simulink model "PassiveHydPTO_Version_3"  (R2014a)
settings: Solver=ode23tb  StartTime=0.0  StopTime=param.stop  FixedStep=0.01  MaxStep=0.05  RelTol=1e-6
values from neighbouring files (symbols this model uses):
  alpha = 1    [Main.m]
  Amax = 0.001    [Main.m]
  Amin = 1e-8    (= 1e-08)    [Main.m]
  Ap = 2.35e-2    (= 0.0235)    [Main.m]
  Beta_e = 1.86e9    (= 1860000000)    [Main.m]
  bf = 0.05*bg    (= 0.118735)    [Main.m]
  bg = 2.3747    [Main.m]
  Cd = 0.61    [Main.m]
  D = 3.9789e-5    (= 3.9789e-05)    [Main.m]
  f = 1/period    (= 0.1)    [Main.m]
  J = 3.961    [Main.m]
  k1 = 200    [Main.m]
  k2 = atanh((Amin-(Amax-Amin)/2)*      2/(Amax - Amin))*1/(pMin-(pMax + pMin)/2)    [Main.m]
  omega_i = 0    [Main.m]
  pAeq = pCeq    (= 21333333.3333)    [Main.m]
  pAi = pAeq    (= 21333333.3333)    [Main.m]
  pAupper_limit = 32e6    (= 32000000)    [Main.m]
  pBeq = pCeq    (= 21333333.3333)    [Main.m]
  pBi = pBeq    (= 21333333.3333)    [Main.m]
  pBupper_limit = 32e6    (= 32000000)    [Main.m]
  pCprecharge = 0.9*pClower_limit    (= 19200000)    [Main.m]
  pDprecharge = 0.9*pDlower_limit    (= 9600000)    [Main.m]
  pMax = 1e6    (= 1000000)    [Main.m]
  pMin = 0.75e6    (= 750000)    [Main.m]
  rho = 850    [Main.m]
  VC0 = 7.5    [Main.m]
  VCeq = VC0*(1-(pCprecharge/pCeq)^(1/1.4))    (= 0.543715404282)    [Main.m]
  VD0 = 3    [Main.m]
  VDeq = VDmax    (= 1.30403881906)    [Main.m]
  Vo = Ap*5    (= 0.1175)    [Main.m]
settings Model: Creator=sor  LastModifiedBy=sor

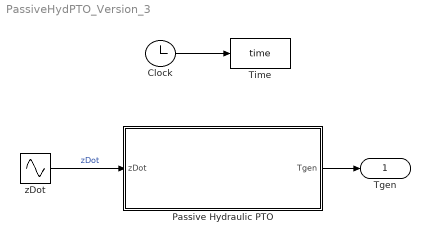
== system PassiveHydPTO_Version_3 ==
  Clock : Clock
  "Passive Hydraulic PTO " : Subsystem
  Time : ToWorkspace  VariableName=time  SampleTime=-1
  zDot : Sin  Amplitude=0.8  Frequency=2*pi*f  SampleTime=0
  Tgen : Outport
  wires:
  Clock/1 -> Time/1
  zDot/1 -> "Passive Hydraulic PTO "/1(zDot)  "zDot"
  "Passive Hydraulic PTO "/1(Tgen) -> Tgen/1

== system PassiveHydPTO_Version_3/Passive Hydraulic PTO  ==
  zDot : Inport
  High Pressure Accumulator : Subsystem
  Low Pressure Accumulator : Subsystem
  Motor Generator : Subsystem
  "Piston Pump " : Subsystem
  Rectified Valve : Subsystem
  Tgen : Outport
  wires:
  "Piston Pump "/1(pA) -> Rectified Valve/1(pA)
  Motor Generator/1(Tgen) -> Tgen/1
  High Pressure Accumulator/1(pC) -> Motor Generator/1(pC), Rectified Valve/3(pC)  "pC"
  Low Pressure Accumulator/1(pD) -> Rectified Valve/4(pD), Motor Generator/2(pD)  "pD"
  "Piston Pump "/2(pB) -> Rectified Valve/2(pB)
  zDot/1 -> "Piston Pump "/1(zDot)
  Rectified Valve/1(Vdot) -> Low Pressure Accumulator/1(Vdot), High Pressure Accumulator/1(Vdot), "Piston Pump "/2(Vdot)
  Motor Generator/2(omega) -> Low Pressure Accumulator/2(omega), High Pressure Accumulator/2(omega)

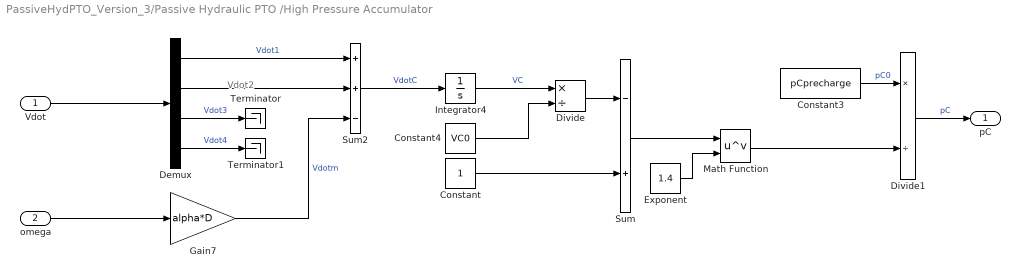
== system PassiveHydPTO_Version_3/Passive Hydraulic PTO /High Pressure Accumulator ==
  note: Vdot2
  Vdot : Inport
  omega : Inport  Port=2
  Constant : Constant
  Constant3 : Constant  Value=pCprecharge
  Constant4 : Constant  Value=VC0
  Demux : Demux
  Divide : Product  Inputs=*/
  Divide1 : Product  Inputs=*/
  Exponent : Constant  Value=1.4
  Gain7 : Gain  Gain=alpha*D
  Integrator4 : Integrator  InitialCondition=VCeq
  Math Function : Math  Operator=pow  SaturateOnIntegerOverflow=on
  Sum : Sum  Inputs=-+
  Sum2 : Sum  Inputs=++-
  Terminator : Terminator
  Terminator1 : Terminator
  pC : Outport
  wires:
  Sum2/1 -> Integrator4/1  "VdotC"
  Integrator4/1 -> Divide/1  "VC"
  Constant4/1 -> Divide/2
  Constant/1 -> Sum/2
  Divide/1 -> Sum/1
  Exponent/1 -> Math Function/2
  Sum/1 -> Math Function/1
  Math Function/1 -> Divide1/2
  Constant3/1 -> Divide1/1  "pC0"
  Divide1/1 -> pC/1  "pC"
  Vdot/1 -> Demux/1
  Demux/3 -> Terminator/1  "Vdot3"
  Demux/4 -> Terminator1/1  "Vdot4"
  omega/1 -> Gain7/1
  Demux/1 -> Sum2/1  "Vdot1"
  Demux/2 -> Sum2/2
  Gain7/1 -> Sum2/3  "Vdotm"

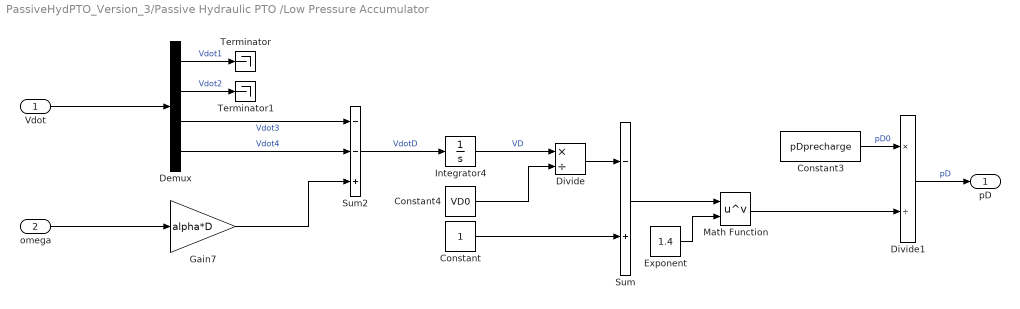
== system PassiveHydPTO_Version_3/Passive Hydraulic PTO /Low Pressure Accumulator ==
  Vdot : Inport
  omega : Inport  Port=2
  Constant : Constant
  Constant3 : Constant  Value=pDprecharge
  Constant4 : Constant  Value=VD0
  Demux : Demux
  Divide : Product  Inputs=*/
  Divide1 : Product  Inputs=*/
  Exponent : Constant  Value=1.4
  Gain7 : Gain  Gain=alpha*D
  Integrator4 : Integrator  InitialCondition=VDeq
  Math Function : Math  Operator=pow  SaturateOnIntegerOverflow=on
  Sum : Sum  Inputs=-+
  Sum2 : Sum  Inputs=--+
  Terminator : Terminator
  Terminator1 : Terminator
  pD : Outport
  wires:
  Sum2/1 -> Integrator4/1  "VdotD"
  Integrator4/1 -> Divide/1  "VD"
  Constant4/1 -> Divide/2
  Constant/1 -> Sum/2
  Divide/1 -> Sum/1
  Exponent/1 -> Math Function/2
  Sum/1 -> Math Function/1
  Math Function/1 -> Divide1/2
  Constant3/1 -> Divide1/1  "pD0"
  Divide1/1 -> pD/1  "pD"
  Vdot/1 -> Demux/1
  Demux/3 -> Sum2/1  "Vdot3"
  Demux/4 -> Sum2/2  "Vdot4"
  omega/1 -> Gain7/1
  Gain7/1 -> Sum2/3
  Demux/1 -> Terminator/1  "Vdot1"
  Demux/2 -> Terminator1/1  "Vdot2"

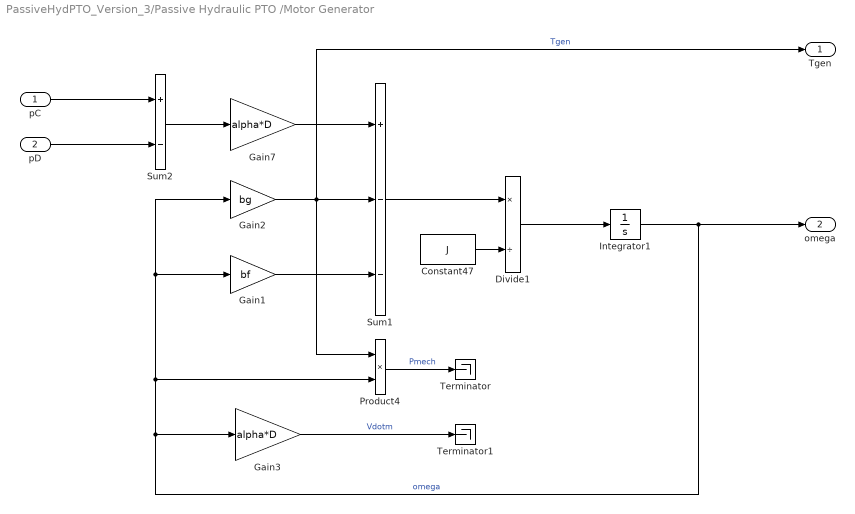
== system PassiveHydPTO_Version_3/Passive Hydraulic PTO /Motor Generator ==
  pC : Inport
  pD : Inport  Port=2
  Constant47 : Constant  Value=J
  Divide1 : Product  Inputs=*/
  Gain1 : Gain  Gain=bf
  Gain2 : Gain  Gain=bg
  Gain3 : Gain  Gain=alpha*D
  Gain7 : Gain  Gain=alpha*D
  Integrator1 : Integrator  InitialCondition=omega_i
  Product4 : Product
  Sum1 : Sum  Inputs=+--
  Sum2 : Sum  Inputs=+-
  Terminator : Terminator
  Terminator1 : Terminator
  Tgen : Outport
  omega : Outport  Port=2
  wires:
  pC/1 -> Sum2/1
  pD/1 -> Sum2/2
  Sum2/1 -> Gain7/1
  Gain7/1 -> Sum1/1
  Gain2/1 -> Product4/1, Tgen/1, Sum1/2  "Tgen"
  Gain1/1 -> Sum1/3
  Sum1/1 -> Divide1/1
  Constant47/1 -> Divide1/2
  Product4/1 -> Terminator/1  "Pmech"
  Divide1/1 -> Integrator1/1
  Integrator1/1 -> Gain3/1, Gain1/1, Gain2/1, Product4/2, omega/1  "omega"
  Gain3/1 -> Terminator1/1  "Vdotm"

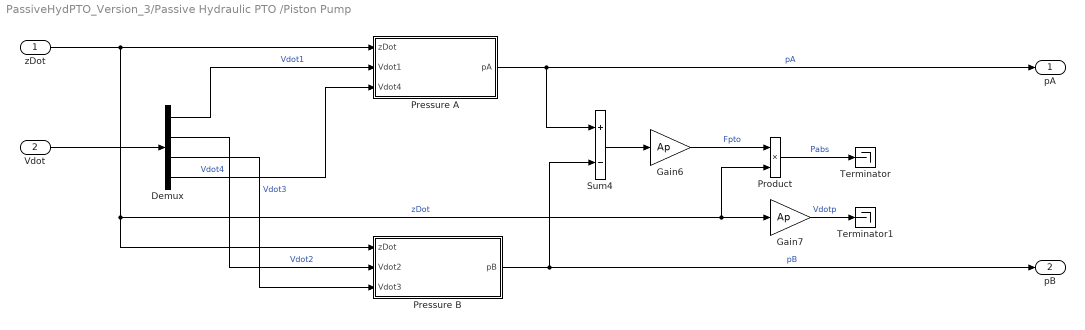
== system PassiveHydPTO_Version_3/Passive Hydraulic PTO /Piston Pump  ==
  zDot : Inport
  Vdot : Inport  Port=2
  Demux : Demux
  Gain6 : Gain  Gain=Ap
  Gain7 : Gain  Gain=Ap
  Pressure A : Subsystem
  Pressure B : Subsystem
  Product : Product
  Sum4 : Sum  Inputs=+-
  Terminator : Terminator
  Terminator1 : Terminator
  pA : Outport
  pB : Outport  Port=2
  wires:
  Pressure A/1(pA) -> pA/1, Sum4/1  "pA"
  Pressure B/1(pB) -> Sum4/2, pB/1  "pB"
  Gain7/1 -> Terminator1/1  "Vdotp"
  Gain6/1 -> Product/1  "Fpto"
  Product/1 -> Terminator/1  "Pabs"
  Vdot/1 -> Demux/1
  zDot/1 -> Gain7/1, Product/2, Pressure B/1(zDot), Pressure A/1(zDot)  "zDot"
  Demux/1 -> Pressure A/2(Vdot1)  "Vdot1"
  Demux/2 -> Pressure B/2(Vdot2)  "Vdot2"
  Demux/3 -> Pressure B/3(Vdot3)  "Vdot3"
  Demux/4 -> Pressure A/3(Vdot4)  "Vdot4"
  Sum4/1 -> Gain6/1

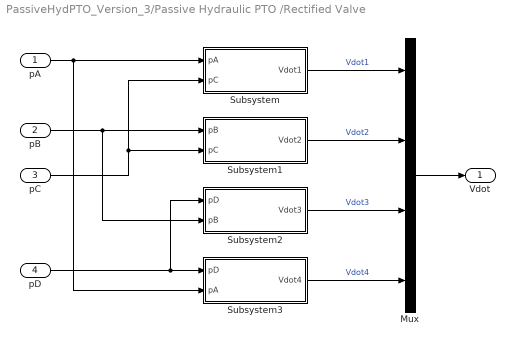
== system PassiveHydPTO_Version_3/Passive Hydraulic PTO /Rectified Valve ==
  pA : Inport
  pB : Inport  Port=2
  pC : Inport  Port=3
  pD : Inport  Port=4
  Mux : Mux
  Subsystem : Subsystem
  Subsystem1 : Subsystem
  Subsystem2 : Subsystem
  Subsystem3 : Subsystem
  Vdot : Outport
  wires:
  pA/1 -> Subsystem3/2(pA), Subsystem/1(pA)
  pB/1 -> Subsystem2/2(pB), Subsystem1/1(pB)
  pC/1 -> Subsystem1/2(pC), Subsystem/2(pC)
  pD/1 -> Subsystem3/1(pD), Subsystem2/1(pD)
  Subsystem3/1(Vdot4) -> Mux/4  "Vdot4"
  Subsystem2/1(Vdot3) -> Mux/3  "Vdot3"
  Subsystem1/1(Vdot2) -> Mux/2  "Vdot2"
  Subsystem/1(Vdot1) -> Mux/1  "Vdot1"
  Mux/1 -> Vdot/1

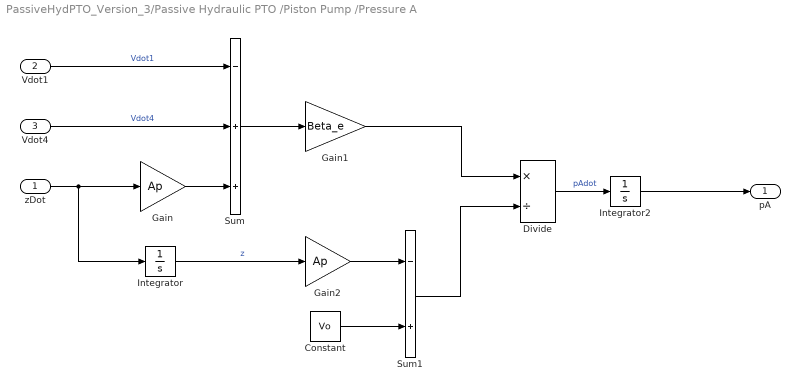
== system PassiveHydPTO_Version_3/Passive Hydraulic PTO /Piston Pump /Pressure A ==
  zDot : Inport
  Vdot1 : Inport  Port=2
  Vdot4 : Inport  Port=3
  Constant : Constant  Value=Vo
  Divide : Product  Inputs=*/
  Gain : Gain  Gain=Ap
  Gain1 : Gain  Gain=Beta_e
  Gain2 : Gain  Gain=Ap
  Integrator : Integrator
  Integrator2 : Integrator  InitialCondition=pAi  UpperSaturationLimit=pAupper_limit  LowerSaturationLimit=pAeq
  Sum : Sum  Inputs=-++
  Sum1 : Sum  Inputs=-+
  pA : Outport
  wires:
  Gain/1 -> Sum/3
  Sum/1 -> Gain1/1
  zDot/1 -> Integrator/1, Gain/1
  Integrator/1 -> Gain2/1  "z"
  Gain2/1 -> Sum1/1
  Constant/1 -> Sum1/2
  Gain1/1 -> Divide/1
  Sum1/1 -> Divide/2
  Vdot1/1 -> Sum/1  "Vdot1"
  Divide/1 -> Integrator2/1  "pAdot"
  Vdot4/1 -> Sum/2  "Vdot4"
  Integrator2/1 -> pA/1

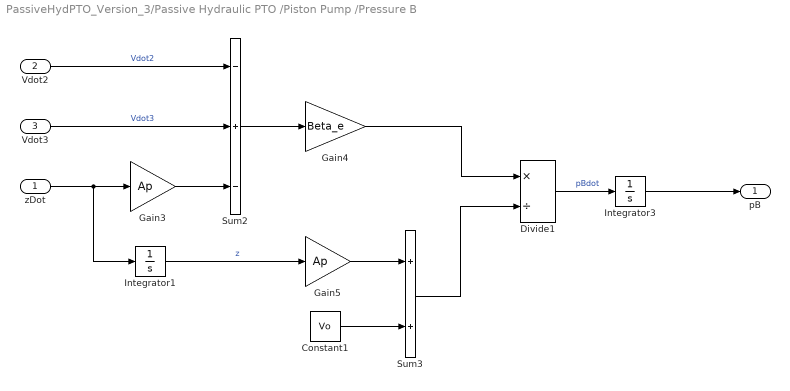
== system PassiveHydPTO_Version_3/Passive Hydraulic PTO /Piston Pump /Pressure B ==
  zDot : Inport
  Vdot2 : Inport  Port=2
  Vdot3 : Inport  Port=3
  Constant1 : Constant  Value=Vo
  Divide1 : Product  Inputs=*/
  Gain3 : Gain  Gain=Ap
  Gain4 : Gain  Gain=Beta_e
  Gain5 : Gain  Gain=Ap
  Integrator1 : Integrator
  Integrator3 : Integrator  InitialCondition=pBi  UpperSaturationLimit=pBupper_limit  LowerSaturationLimit=pBeq
  Sum2 : Sum  Inputs=-+-
  Sum3 : Sum
  pB : Outport
  wires:
  Gain3/1 -> Sum2/3
  Sum2/1 -> Gain4/1
  zDot/1 -> Integrator1/1, Gain3/1
  Integrator1/1 -> Gain5/1  "z"
  Gain5/1 -> Sum3/1
  Constant1/1 -> Sum3/2
  Gain4/1 -> Divide1/1
  Sum3/1 -> Divide1/2
  Divide1/1 -> Integrator3/1  "pBdot"
  Vdot2/1 -> Sum2/1  "Vdot2"
  Vdot3/1 -> Sum2/2  "Vdot3"
  Integrator3/1 -> pB/1

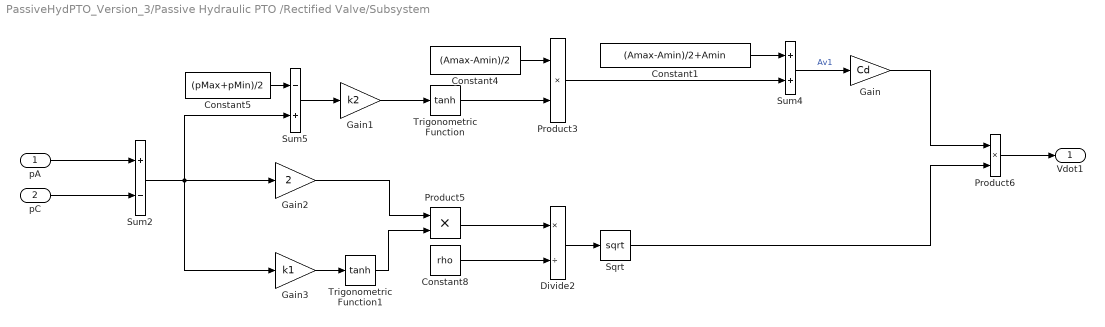
== system PassiveHydPTO_Version_3/Passive Hydraulic PTO /Rectified Valve/Subsystem ==
  pA : Inport
  pC : Inport  Port=2
  Constant1 : Constant  Value=(Amax-Amin)/2+Amin
  Constant4 : Constant  Value=(Amax-Amin)/2
  Constant5 : Constant  Value=(pMax+pMin)/2
  Constant8 : Constant  Value=rho
  Divide2 : Product  Inputs=*/
  Gain : Gain  Gain=Cd
  Gain1 : Gain  Gain=k2
  Gain2 : Gain  Gain=2
  Gain3 : Gain  Gain=k1
  Product3 : Product
  Product5 : Product
  Product6 : Product
  Sqrt : Sqrt  SaturateOnIntegerOverflow=on
  Sum2 : Sum  Inputs=+-
  Sum4 : Sum
  Sum5 : Sum  Inputs=-+
  Trigonometric Function : Trigonometry  Operator=tanh
  Trigonometric Function1 : Trigonometry  Operator=tanh
  Vdot1 : Outport
  wires:
  Gain1/1 -> Trigonometric Function/1
  Trigonometric Function/1 -> Product3/2
  Product3/1 -> Sum4/2
  Sum5/1 -> Gain1/1
  Sum4/1 -> Gain/1  "Av1"
  Gain3/1 -> Trigonometric Function1/1
  Gain2/1 -> Product5/1
  Trigonometric Function1/1 -> Product5/2
  Sqrt/1 -> Product6/2
  Gain/1 -> Product6/1
  Constant8/1 -> Divide2/2
  Product5/1 -> Divide2/1
  Divide2/1 -> Sqrt/1
  pA/1 -> Sum2/1
  pC/1 -> Sum2/2
  Product6/1 -> Vdot1/1
  Constant4/1 -> Product3/1
  Constant5/1 -> Sum5/1
  Constant1/1 -> Sum4/1
  Sum2/1 -> Gain3/1, Sum5/2, Gain2/1

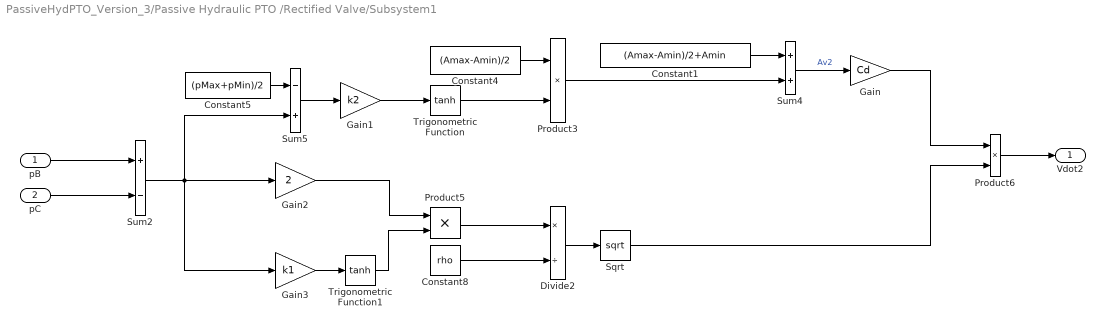
== system PassiveHydPTO_Version_3/Passive Hydraulic PTO /Rectified Valve/Subsystem1 ==
  pB : Inport
  pC : Inport  Port=2
  Constant1 : Constant  Value=(Amax-Amin)/2+Amin
  Constant4 : Constant  Value=(Amax-Amin)/2
  Constant5 : Constant  Value=(pMax+pMin)/2
  Constant8 : Constant  Value=rho
  Divide2 : Product  Inputs=*/
  Gain : Gain  Gain=Cd
  Gain1 : Gain  Gain=k2
  Gain2 : Gain  Gain=2
  Gain3 : Gain  Gain=k1
  Product3 : Product
  Product5 : Product
  Product6 : Product
  Sqrt : Sqrt  SaturateOnIntegerOverflow=on
  Sum2 : Sum  Inputs=+-
  Sum4 : Sum
  Sum5 : Sum  Inputs=-+
  Trigonometric Function : Trigonometry  Operator=tanh
  Trigonometric Function1 : Trigonometry  Operator=tanh
  Vdot2 : Outport
  wires:
  Gain1/1 -> Trigonometric Function/1
  Trigonometric Function/1 -> Product3/2
  Product3/1 -> Sum4/2
  Sum5/1 -> Gain1/1
  Sum4/1 -> Gain/1  "Av2"
  Gain3/1 -> Trigonometric Function1/1
  Gain2/1 -> Product5/1
  Trigonometric Function1/1 -> Product5/2
  Sqrt/1 -> Product6/2
  Gain/1 -> Product6/1
  Constant8/1 -> Divide2/2
  Product5/1 -> Divide2/1
  Divide2/1 -> Sqrt/1
  pB/1 -> Sum2/1
  pC/1 -> Sum2/2
  Product6/1 -> Vdot2/1
  Constant4/1 -> Product3/1
  Constant5/1 -> Sum5/1
  Constant1/1 -> Sum4/1
  Sum2/1 -> Gain3/1, Sum5/2, Gain2/1

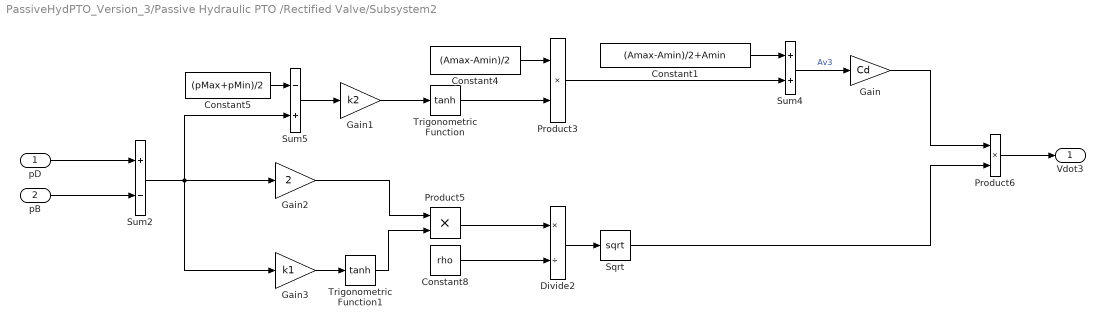
== system PassiveHydPTO_Version_3/Passive Hydraulic PTO /Rectified Valve/Subsystem2 ==
  pD : Inport
  pB : Inport  Port=2
  Constant1 : Constant  Value=(Amax-Amin)/2+Amin
  Constant4 : Constant  Value=(Amax-Amin)/2
  Constant5 : Constant  Value=(pMax+pMin)/2
  Constant8 : Constant  Value=rho
  Divide2 : Product  Inputs=*/
  Gain : Gain  Gain=Cd
  Gain1 : Gain  Gain=k2
  Gain2 : Gain  Gain=2
  Gain3 : Gain  Gain=k1
  Product3 : Product
  Product5 : Product
  Product6 : Product
  Sqrt : Sqrt  SaturateOnIntegerOverflow=on
  Sum2 : Sum  Inputs=+-
  Sum4 : Sum
  Sum5 : Sum  Inputs=-+
  Trigonometric Function : Trigonometry  Operator=tanh
  Trigonometric Function1 : Trigonometry  Operator=tanh
  Vdot3 : Outport
  wires:
  Gain1/1 -> Trigonometric Function/1
  Trigonometric Function/1 -> Product3/2
  Product3/1 -> Sum4/2
  Sum5/1 -> Gain1/1
  Sum4/1 -> Gain/1  "Av3"
  Gain3/1 -> Trigonometric Function1/1
  Gain2/1 -> Product5/1
  Trigonometric Function1/1 -> Product5/2
  Sqrt/1 -> Product6/2
  Gain/1 -> Product6/1
  Constant8/1 -> Divide2/2
  Product5/1 -> Divide2/1
  Divide2/1 -> Sqrt/1
  pD/1 -> Sum2/1
  pB/1 -> Sum2/2
  Product6/1 -> Vdot3/1
  Constant4/1 -> Product3/1
  Constant5/1 -> Sum5/1
  Constant1/1 -> Sum4/1
  Sum2/1 -> Gain3/1, Sum5/2, Gain2/1

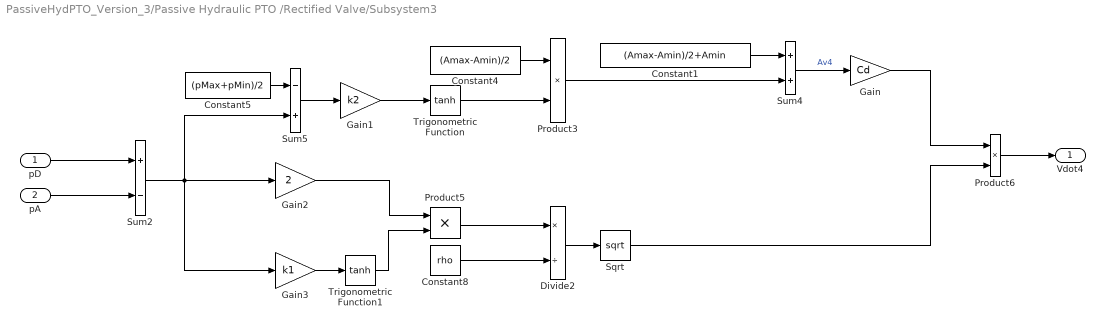
== system PassiveHydPTO_Version_3/Passive Hydraulic PTO /Rectified Valve/Subsystem3 ==
  pD : Inport
  pA : Inport  Port=2
  Constant1 : Constant  Value=(Amax-Amin)/2+Amin
  Constant4 : Constant  Value=(Amax-Amin)/2
  Constant5 : Constant  Value=(pMax+pMin)/2
  Constant8 : Constant  Value=rho
  Divide2 : Product  Inputs=*/
  Gain : Gain  Gain=Cd
  Gain1 : Gain  Gain=k2
  Gain2 : Gain  Gain=2
  Gain3 : Gain  Gain=k1
  Product3 : Product
  Product5 : Product
  Product6 : Product
  Sqrt : Sqrt  SaturateOnIntegerOverflow=on
  Sum2 : Sum  Inputs=+-
  Sum4 : Sum
  Sum5 : Sum  Inputs=-+
  Trigonometric Function : Trigonometry  Operator=tanh
  Trigonometric Function1 : Trigonometry  Operator=tanh
  Vdot4 : Outport
  wires:
  Gain1/1 -> Trigonometric Function/1
  Trigonometric Function/1 -> Product3/2
  Product3/1 -> Sum4/2
  Sum5/1 -> Gain1/1
  Sum4/1 -> Gain/1  "Av4"
  Gain3/1 -> Trigonometric Function1/1
  Gain2/1 -> Product5/1
  Trigonometric Function1/1 -> Product5/2
  Sqrt/1 -> Product6/2
  Gain/1 -> Product6/1
  Constant8/1 -> Divide2/2
  Product5/1 -> Divide2/1
  Divide2/1 -> Sqrt/1
  pD/1 -> Sum2/1
  pA/1 -> Sum2/2
  Product6/1 -> Vdot4/1
  Constant4/1 -> Product3/1
  Constant5/1 -> Sum5/1
  Constant1/1 -> Sum4/1
  Sum2/1 -> Gain3/1, Sum5/2, Gain2/1
